simulink model "SimCodeGen_mfun_model"  (R2023a)
settings: Solver=VariableStepAuto  StartTime=0.0  StopTime=10.0  RelTol=1e-3
values from neighbouring files (symbols this model uses):
  x1_ic = zeros(6,1)    [init_Catalyst_5.m]
undefined symbols (not defined in the file or in its folder): params_CRS
settings Model: Creator=Flo  LastModifiedBy=Flo

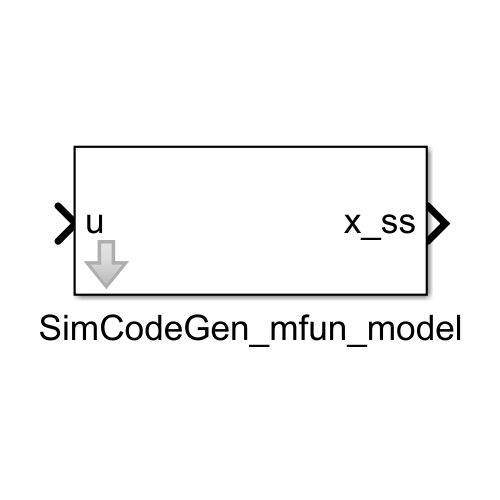
[thumbnail: Simulink's stored preview of the top-level diagram]
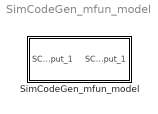
== system SimCodeGen_mfun_model ==
  SimCodeGen_mfun_model : Subsystem  mask{SC_param_0=params_CRS, SC_x1_ic=x1_ic}
      mask prompts: SC_param_0 "params_CRS"
      mask Display:
      | port_label('input', 1, 'u');
      | port_label('output', 1, 'x_ss');

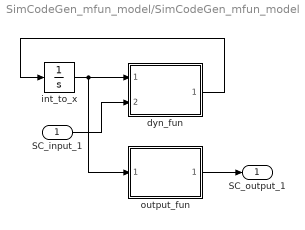
== system SimCodeGen_mfun_model/SimCodeGen_mfun_model ==
  SC_input_1 : Inport
  dyn_fun : MATLAB Function  TreatAsAtomicUnit=on
  int_to_x : Integrator  InitialCondition=[SC_x1_ic]
  output_fun : MATLAB Function  TreatAsAtomicUnit=on
  SC_output_1 : Outport
  wires:
  output_fun/1(SC_output_0) -> SC_output_1/1
  int_to_x/1 -> output_fun/1(SC_state), dyn_fun/1(SC_state)
  SC_input_1/1 -> dyn_fun/2(SC_input_0)
  dyn_fun/1(SC_state_dot) -> int_to_x/1

== matlab function SimCodeGen_mfun_model/dyn_fun ==
  data: SC_state input size=[6]; SC_state_dot output size=[6]; SC_input_0 input size=[3]; SC_param_0 parameter
function SC_state_dot  = dyn_fun(SC_state, SC_input_0, SC_param_0)
    SC_state_dot = zeros(6, 1);
    SC_state_x_0 = SC_state(1:6);
    SC_eval = zeros(6,1);
    SC_eval(1) = SC_state_x_0(4);
    SC_eval(2) = SC_state_x_0(5);
    SC_eval(3) = SC_state_x_0(6);
    t1 = SC_state_x_0(3);
    t2 = cos(t1);
    t3 = t2 ^ 2;
    t4 = SC_param_0(3);
    t6 = SC_param_0(5);
    t7 = t6 ^ 2;
    t9 = SC_param_0(6);
    t10 = t9 * t4;
    t11 = t2 * t6;
    t12 = SC_state_x_0(2);
    t13 = sin(t12);
    t17 = t13 ^ 2;
    t18 = t9 ^ 2;
    t21 = SC_param_0(2);
    t23 = SC_param_0(4);
    t24 = t23 ^ 2;
    t26 = SC_param_0(9);
    t27 = cos(t12);
    t28 = t27 ^ 2;
    t30 = SC_param_0(12);
    t31 = sin(t1);
    t32 = t31 ^ 2;
    t34 = SC_param_0(15);
    t35 = t34 ^ 2;
    t38 = SC_param_0(10);
    t40 = SC_param_0(13);
    t48 = t24 * t21;
    t49 = t18 * t4;
    t50 = t48 + t49 - t26 + t38;
    t56 = t4 * t6;
    t58 = t7 * t4;
    t59 = t58 - t30 + t40;
    t14 = SC_eval(1);
    t15 = SC_eval(2);
    t41 = SC_eval(3);
    t53 = t18 * t4;
    t55 = t24 * t21;
    t60 = t7 * t4;
    SC_eval(4) = 0.1e1 / (0.2e1 * t10 * t11 * t13 + t17 * t38 + t17 * t53 + t17 * t55 + t26 * t28 + t3 * t40 + t3 * t60 + t30 * t32 + t35 * SC_param_0(18) + SC_param_0(8)) * (t34 * SC_input_0(1) - 0.2e1 * ((t11 * t10 + t13 * t50) * t15 * t27 - t41 * (t13 * t56 * t9 + t2 * t59) * t31) * t14);
    t68 = SC_param_0(17);
    t69 = t68 ^ 2;
    t70 = SC_param_0(20);
    t71 = t70 * t69;
    t72 = SC_param_0(14);
    t74 = t1 + t12;
    t75 = sin(t74);
    t76 = t75 ^ 2;
    t78 = t4 ^ 2;
    t81 = SC_param_0(19);
    t83 = SC_param_0(16);
    t84 = t83 ^ 2;
    t87 = t81 * t84;
    t98 = SC_param_0(11);
    t80 = t7 * t78;
    t108 = t21 * t24 * t4 * t7 + t69 * t70 * t81 * t84 - t18 * t76 * t80 + t69 * t70 * t98 + t72 * t81 * t84 + t18 * t80 + t48 * t71 + t49 * t71 + t53 * t72 + t55 * t72 + t58 * t87 + t60 * t98 + t72 * t98;
    t109 = 0.1e1 / t108;
    t113 = t14 ^ 2;
    t116 = cos(-t1 + t12);
    t119 = t116 * t113 * t9 * t56 / 0.2e1;
    t122 = sin(0.2e1 * t12);
    t125 = t41 ^ 2;
    t129 = cos(t74);
    t133 = SC_param_0(1);
    t138 = t83 * SC_input_0(2) + t119 + t122 * t50 * t113 / 0.2e1 + t129 * (t113 + 0.2e1 * t125) * t6 * t10 / 0.2e1 + t13 * (t21 * t23 + t10) * t133;
    t140 = t75 * t56;
    t141 = t109 * t9;
    t146 = sin(0.2e1 * t1);
    t149 = t15 ^ 2;
    t158 = t68 * SC_input_0(3) - t119 - t146 * t59 * t113 / 0.2e1 - t6 * t4 * (-t129 * t9 * (t149 + t113 / 0.2e1) + t133 * t2);
    SC_eval(5) = t138 * t109 * (t58 + t71 + t72) + t158 * t141 * t140;
    SC_eval(6) = t138 * t141 * t140 + t158 * t109 * (t48 + t49 + t87 + t98);
    SC_state_dot(1:6) = SC_eval(1:6);
end

== matlab function SimCodeGen_mfun_model/output_fun ==
  data: SC_state input size=[6]; SC_output_0 output size=[6]; SC_param_0 parameter size=[20]
function SC_output_0  = y_fun(SC_state, SC_param_0)
    SC_output_0 = zeros(6,1);
    SC_state_x_0 = SC_state(1:6);
    SC_output_0(1) = SC_state_x_0(1);
    SC_output_0(2) = SC_state_x_0(2);
    SC_output_0(3) = SC_state_x_0(3);
    SC_output_0(4) = SC_state_x_0(4);
    SC_output_0(5) = SC_state_x_0(5);
    SC_output_0(6) = SC_state_x_0(6);
end
